simulink model "C3_1_LiftLoop_step0"  (R2022a)
settings: Solver=VariableStepAuto  StartTime=0.0  StopTime=10.0  RelTol=1e-3
libraries: fl_lib x10, nesl_utility x5, SimscapeFluids_lib x3
settings Model: Creator=amyyang  LastModifiedBy=amyyang
settings SimscapeCC: SimscapeLogType=all  SimscapeLogLimitData=off

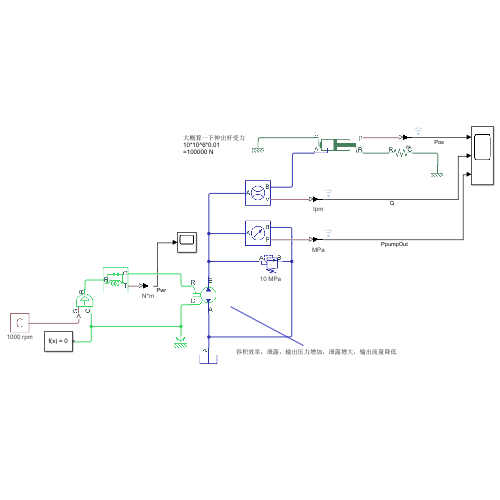
[thumbnail: Simulink's stored preview of the top-level diagram]
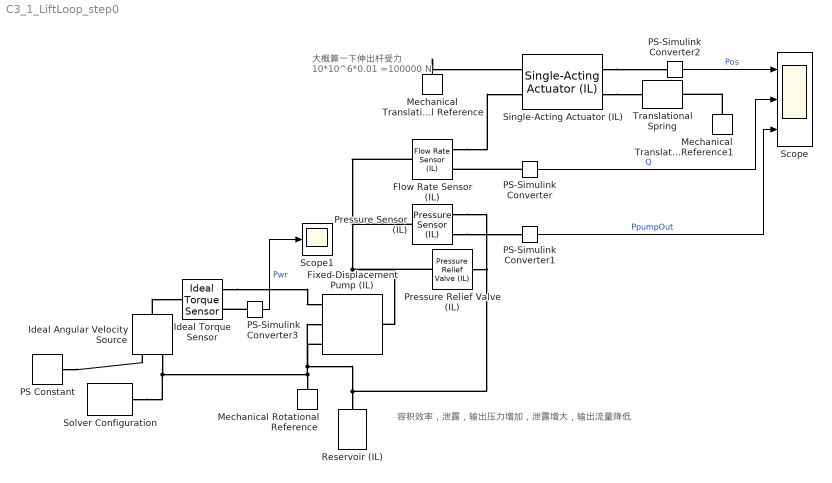
== system C3_1_LiftLoop_step0 ==
  note: 容积效率，泄露，输出压力增加，泄露增大，输出流量降低
  note: 大概算一下伸出杆受力
      | 10*10^6*0.01
      | =100000 N
  Fixed-Displacement Pump (IL) : SimscapeFluids_lib/Isothermal Liquid/Pumps & Motors/Fixed-Displacement Pump (IL)  leakage_friction_spec=fluids.isothermal_liquid.pumps_motors.enum.pump_motor_loss_spec.analytical  displacement=0.1 l/rev  omega_nominal=1000 rpm  p_nominal=10 MPa  vol_eff_nominal=0.92  mech_eff_nominal=0.88  no_load_torque=0 N*m  p_diff_eff_TLU=[.1, 1, 2] MPa  omega_eff_TLU=[25, 50, 100, 200, 300, 400] rad/s  vol_eff_TLU=[.816, .908, .954, .977, .981, .984; .325, .663, .831, .916, .925, .946; .137, .568, .78, .892, .893, .91]  mech_eff_TLU=[.996, .996, .996, .996, .996, .996; .988, .989, .989, .989, .989, .99; .981, .981, .982, .982, .983, .984]  p_diff_loss_TLU=[.1, 1, 2] MPa  omega_loss_TLU=[25, 50, 100, 200, 300, 400] rad/s  vol_loss_TLU=1e-3 * [.023, .023, .023, .023, .0285, .032; .0844, .0842, .0845, .084, .1125, .108; .1079, .108, .11, .108, .1605, .18] m^3/s  mech_loss_TLU=[.002, .002, .002, .002, .002, .002; .0607, .0556, .0556, .0556, .0556, .0505; .1937, .1937, .1833, .1833, .1729, .1626] N*m  vol_eff_min=1e-3  vol_eff_max=1  mech_eff_min=1e-3  mech_eff_max=1  pressure_threshold=1e-3 MPa  omega_threshold=10 rad/s  quadrant_check=simscape.enum.assert.action.none  pump_mode_check=simscape.enum.assert.action.none  pressure_check=simscape.enum.assert.action.none  p_min_valid=0.101325 MPa
      settings: SourceProductBaseCode=SH  InternalSimscapePortConfiguration="{\"Bottom\":[{\"id\":\"A\",\"label\":\"A\",\"type\":\"foundation.isothermal_liquid.isothermal_liquid\"}],\"Left\":[],\"Right\":[{\"id\":\"R\",\"label\":\"R\",\"type\":\"foundation.mechanical.rotational.rotational\"},{\"id\":\"C\",\"label\":\"C\",\"type\":\"foundation.mechanical.rotational.rotational\"}],\"Top\":[{\"id\":\"B\",\"label\":\"B\",\"type\":\"foundation.isothermal_liquid.isothermal_liquid\"}]}"
  Flow Rate Sensor (IL) : fl_lib/Isothermal Liquid/Sensors/Flow Rate Sensor (IL)  sensor_type=foundation.enum.mass_volumetric_sensor.volumetric
      settings: SourceProductBaseCode=PW,SS,VE  InternalSimscapePortConfiguration="{\"Bottom\":[],\"Left\":[{\"id\":\"A\",\"label\":\"A\",\"type\":\"foundation.isothermal_liquid.isothermal_liquid\"}],\"Right\":[{\"id\":\"B\",\"label\":\"B\",\"type\":\"foundation.isothermal_liquid.isothermal_liquid\"},{\"id\":\"V\",\"label\":\"V\",\"type\":\"output\"}],\"Top\":[]}"
  Ideal Angular Velocity Source : fl_lib/Mechanical/Mechanical Sources/Ideal Angular Velocity Source
      settings: SourceProductBaseCode=PW,SS,VE
  Ideal Torque Sensor : fl_lib/Mechanical/Mechanical Sensors/Ideal Torque Sensor
      settings: SourceProductBaseCode=PW,SS,VE
  Mechanical Rotational Reference : fl_lib/Mechanical/Rotational Elements/Mechanical Rotational Reference
      settings: SourceProductBaseCode=PW,SS,VE
  Mechanical Translational Reference : fl_lib/Mechanical/Translational Elements/Mechanical Translational Reference
      settings: SourceProductBaseCode=PW,SS,VE
  Mechanical Translational Reference1 : fl_lib/Mechanical/Translational Elements/Mechanical Translational Reference
      settings: SourceProductBaseCode=PW,SS,VE
  PS Constant : fl_lib/Physical Signals/Sources/PS Constant  constant=1000 rpm
      settings: AttributesFormatString=%<constant> %<constant_unit>  SourceProductBaseCode=PW,SS,VE
  PS-Simulink Converter : nesl_utility/PS-Simulink Converter  PhysicalDomain=network_engine_domain  SubClassName=ps_output  LeftPortType=input  RightPortType=output  PseudoPeriodic=off  Frequencies=[]  VectorFormat=inherit  Unit=lpm  AffineConversion=off
      settings: SourceProductBaseCode=SS,PW,VE
  PS-Simulink Converter1 : nesl_utility/PS-Simulink Converter  PhysicalDomain=network_engine_domain  SubClassName=ps_output  LeftPortType=input  RightPortType=output  PseudoPeriodic=off  Frequencies=[]  VectorFormat=inherit  Unit=MPa  AffineConversion=off
      settings: SourceProductBaseCode=SS,PW,VE
  PS-Simulink Converter2 : nesl_utility/PS-Simulink Converter  PhysicalDomain=network_engine_domain  SubClassName=ps_output  LeftPortType=input  RightPortType=output  PseudoPeriodic=off  Frequencies=[]  VectorFormat=inherit  Unit=m  AffineConversion=off
      settings: SourceProductBaseCode=SS,PW,VE
  PS-Simulink Converter3 : nesl_utility/PS-Simulink Converter  PhysicalDomain=network_engine_domain  SubClassName=ps_output  LeftPortType=input  RightPortType=output  PseudoPeriodic=off  Frequencies=[]  VectorFormat=inherit  Unit=N*m  AffineConversion=off
      settings: SourceProductBaseCode=SS,PW,VE
  Pressure Relief Valve (IL) : SimscapeFluids_lib/Isothermal Liquid/Valves & Orifices/Pressure Control Valves/Pressure Relief Valve (IL)  set_pressure_spec=foundation.enum.constant_controlled.constant  opening_spec=fluids.isothermal_liquid.valves_orifices.enum.PressureOpeningSpec.Linear  pressure_spec=fluids.isothermal_liquid.valves_orifices.enum.pressure_control_spec.dp  p_set_gauge=0.1 MPa  p_set_differential=10 MPa  p_range=0.1 MPa  area_max=1e-4 m^2  area_leak=1e-10 m^2  p_diff_TLU=[0.2 : 0.2 : 1.2] MPa  p_gauge_TLU=[0.2 : 0.2 : 1.2] MPa  valve_area_TLU=[1e-10, 2e-06, 4e-06, 6e-06, 8e-06, 1e-05] m^2  vol_flow_TLU=[1e-09, 3.6e-05, 8.9e-05, .00015, .00023, .00031] m^3/s  area=inf m^2  Cd=0.64  Re_c=150  smoothing_factor=0.01  pressure_recovery=simscape.enum.onoff.off  opening_dynamics=simscape.enum.onoff.off  tau=0.1 s  enable_faults=simscape.enum.onoff.off  fault_type=fluids.enum.FaultOpening.Closed  fault_trigger=foundation.enum.faultSpec.Temporal  fault_time=5 s
      settings: AttributesFormatString=%<p_set_differential> %<p_set_differential_unit>  SourceProductBaseCode=SH  InternalSimscapePortConfiguration="{\"Bottom\":[],\"Left\":[{\"id\":\"A\",\"label\":\"A\",\"type\":\"foundation.isothermal_liquid.isothermal_liquid\"}],\"Right\":[{\"id\":\"B\",\"label\":\"B\",\"type\":\"foundation.isothermal_liquid.isothermal_liquid\"}],\"Top\":[]}"
  Pressure Sensor (IL) : fl_lib/Isothermal Liquid/Sensors/Pressure Sensor (IL)  pressure_measure=foundation.enum.pressure_measure.difference
      settings: SourceProductBaseCode=PW,SS,VE  InternalSimscapePortConfiguration="{\"Bottom\":[],\"Left\":[{\"id\":\"A\",\"label\":\"A\",\"type\":\"foundation.isothermal_liquid.isothermal_liquid\"}],\"Right\":[{\"id\":\"B\",\"label\":\"B\",\"type\":\"foundation.isothermal_liquid.isothermal_liquid\"},{\"id\":\"P\",\"label\":\"P\",\"type\":\"output\"}],\"Top\":[]}"
  Reservoir (IL) : fl_lib/Isothermal Liquid/Elements/Reservoir (IL)  reservoir_type=foundation.enum.constant_controlled.constant  pressure_spec=foundation.enum.pressure_spec.atmospheric  reservoir_pressure=0.101325 MPa
      settings: SourceProductBaseCode=PW,SS,VE
  Scope : Scope  NumInputPorts=3
  Scope1 : Scope
  Single-Acting Actuator (IL) : SimscapeFluids_lib/Isothermal Liquid/Actuators/Single-Acting Actuator (IL)  mech_orientation=foundation.enum.MechOrientationTranslational.Positive  piston_area=0.01 m^2  stroke=1 m  dead_volume=1e-5 m^3  pressure_spec=foundation.enum.pressure_spec.atmospheric  environment_pressure=0.101325 MPa  stiff_coeff=1e12 N/m  damping_coeff=150 N*s/m  hardstop_model=simscape.enum.hardstop.smooth  transition=0.1 mm  cushion_spec=simscape.enum.onoff.off  area_plunger=1e-4 m^2  length_plunger=1e-3 m  area_cushion_orifice=1e-6 m^2  area_leak_plunger=1e-7 m^2  p_crack_differential=0.01 MPa  press_max_differential=0.1 MPa  check_valve_area_max=1e-4 m^2  check_valve_area_leak=1e-10 m^2  smoothing_factor=0.01  friction_spec=simscape.enum.onoff.off  breakaway_Coulomb_ratio=1.2  breakaway_velocity=0.1 m/s  preload_force=20 N  Coulomb_coeff=1e-6 N/Pa  viscous_coeff=100 N*s/m  leakage_spec=simscape.enum.onoff.off  clearance=1e-4 m  piston_length=0.01 m  displacement_spec=foundation.enum.DisplacementSpec.Calculate  x0=0 m  dynamic_compressibility=simscape.enum.onoff.on  p0=0.101325 MPa
      settings: SourceProductBaseCode=SH  InternalSimscapePortConfiguration="{\"Bottom\":[],\"Left\":[{\"id\":\"C\",\"label\":\"C\",\"type\":\"foundation.mechanical.translational.translational\"},{\"id\":\"A\",\"label\":\"A\",\"type\":\"foundation.isothermal_liquid.isothermal_liquid\"}],\"Right\":[{\"id\":\"p_out\",\"label\":\"p\",\"type\":\"output\"},{\"id\":\"R\",\"label\":\"R\",\"type\":\"foundation.mechanical.translational.translational\"}],\"Top\":[]}"
  Solver Configuration : nesl_utility/Solver Configuration  PhysicalDomain=network_engine_domain  SubClassName=solver  LeftPortType=input  RightPortType=generic  Tones=[]  Harmonics=[]  SimulateNoise=off  Profile=off  UseLocalSampling=off  EnableSwitchedLinearOptims=on  FrequencyDomain=off  UseCCode=off  RelTol=0.001  AbsTol=0.001  MinStep=1e-09  ToWorkspace=off  RevertToSquareIcSolve=off  NumHomotopyIterations=100  PhasorMode=off  PhasorModeNumHarmonics=1  IndexReductionMethod=DerivativeReplacement  DoDC=off  ResidualTolerance=1e-09  UseLocalSolver=off  LocalSolverChoice=NE_BACKWARD_EULER_ADVANCER  LocalSolverSampleTime=0.001  DoFixedCost=off  MaxNonlinIter=3  MaxModeIter=2  ComputeImpulses=off  ImpulseIterations=2  LinearAlgebra=auto  LinearAlgebraNumThread=0  EquationFormulation=NE_TIME_EF  DelaysMemoryBudget=1024  AutomaticFiltering=on  FilteringTimeConstant=0.001  PartitionStorageMethod=AS_NEEDED  PartitionMemoryBudget=1024  PartitionMethod=ROBUST
      settings: SourceProductBaseCode=SS,PW,VE
  Translational Spring : fl_lib/Mechanical/Translational Elements/Translational Spring  spr_rate=10^5 N/m  v_specify=off  v_priority=None  v=0 m/s  v_nominal_specify=off  v_nominal_unit=m/s  v_nominal_value=1  f_specify=off  f_priority=None  f=0 N  f_nominal_specify=off  f_nominal_unit=N  f_nominal_value=1  x_specify=off  x_priority=High  x=0 m  x_nominal_specify=off  x_nominal_unit=m  x_nominal_value=1
      settings: SourceProductBaseCode=PW,SS,VE
  wires:
  PS-Simulink Converter/1 -> Scope/2  "Q"
  PS-Simulink Converter1/1 -> Scope/3  "PpumpOut"
  PS-Simulink Converter2/1 -> Scope/1  "Pos"
  PS-Simulink Converter3/1 -> Scope1/1  "Pwr"
  connections:
  Ideal Angular Velocity Source/RConn2 -- Solver Configuration/RConn1 -- Fixed-Displacement Pump (IL)/RConn2 -- Mechanical Rotational Reference/LConn1
  Fixed-Displacement Pump (IL)/RConn3 -- Pressure Relief Valve (IL)/RConn1 -- Pressure Sensor (IL)/RConn1 -- Reservoir (IL)/LConn1
  Ideal Angular Velocity Source/LConn1 -- Ideal Torque Sensor/LConn1
  PS Constant/RConn1 -- Ideal Angular Velocity Source/RConn1
  Pressure Relief Valve (IL)/LConn1 -- Pressure Sensor (IL)/LConn1 -- Flow Rate Sensor (IL)/LConn1 -- Fixed-Displacement Pump (IL)/LConn1
  PS-Simulink Converter/LConn1 -- Flow Rate Sensor (IL)/RConn2
  Mechanical Translational Reference/LConn1 -- Single-Acting Actuator (IL)/LConn1
  Single-Acting Actuator (IL)/RConn2 -- Translational Spring/LConn1
  Mechanical Translational Reference1/LConn1 -- Translational Spring/RConn1
  Flow Rate Sensor (IL)/RConn1 -- Single-Acting Actuator (IL)/LConn2
  Pressure Sensor (IL)/RConn2 -- PS-Simulink Converter1/LConn1
  Single-Acting Actuator (IL)/RConn1 -- PS-Simulink Converter2/LConn1
  Ideal Torque Sensor/RConn1 -- Fixed-Displacement Pump (IL)/RConn1
  PS-Simulink Converter3/LConn1 -- Ideal Torque Sensor/RConn2
